simulink model "gm_CustArch_v13_vnl"  (R2020a)
settings: Solver=FixedStepDiscrete  StartTime=0.0  StopTime=840000  RelTol=1e-3
libraries: simulink x185, hdlsllib x109, hdlmdlgenlib x25, dsparch4 x1
(part 3 of 4)

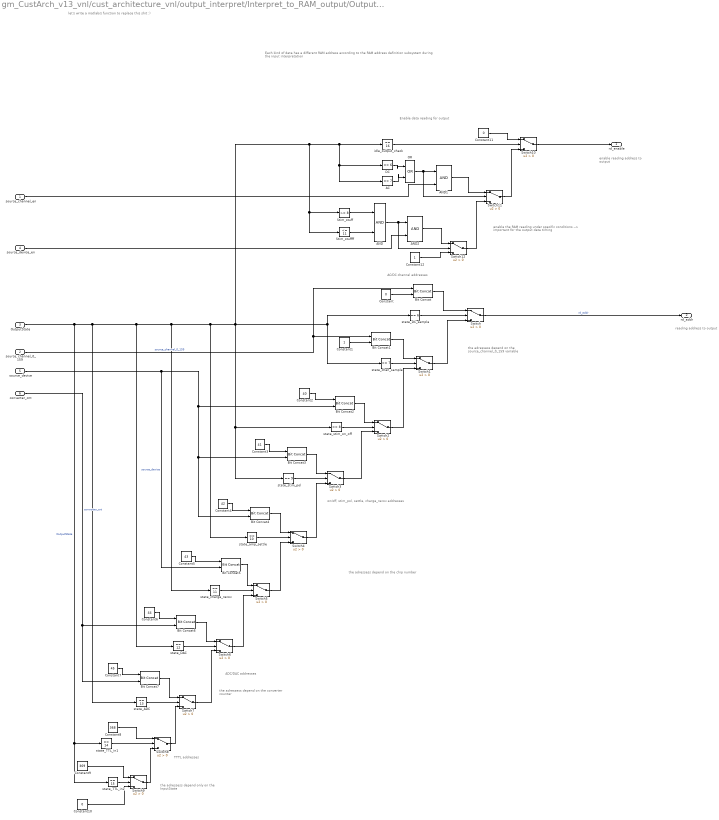
== system gm_CustArch_v13_vnl/cust_architecture_vnl/output_interpret/Interpret_to_RAM_output/Output_State_to_RAM_address (to read) ==
  note: enable reading address
      | to output
  note: Each kind of data has a different RAM
      | address according to the
      | RAM address definition subsystem during the
      | input interpretation
  note: the adressess depend on the
      | source_channel_0_159 variable
  note: AC/DC channel addresses
  note: ADC/DAC addresses
  note: on/off, stim_pol, settle, charge_recov addresses
  note: the adressess depend on the converter
      | counter
  note: the adressess depend only on the
      | InputState
  note: the adressess depend on the chip number
  note: TTTL addresses
  note: let's write a matlab/s function to replace this shit :)
  note: Enable data reading for output
  note: enable the RAM reading under specific conditions
      | --> important for the output data timing
  note: reading address
      | to output
  source_channel_en : Inport
  source_channel_0_159 : Inport  Port=2
  OutputState : Inport  Port=3
  source_device_en : Inport  Port=4
  source_device : Inport  Port=5
  converter_cnt : Inport  Port=6
  AC : simulink/Logic and Bit Operations/Compare To Constant  relop===  const=7  OutDataTypeStr=boolean
  AND : Logic  IconShape=distinctive  AllPortsSameDT=off  OutDataTypeStr=boolean
  AND1 : Logic  IconShape=distinctive  AllPortsSameDT=off  OutDataTypeStr=boolean
  AND2 : Logic  IconShape=distinctive  AllPortsSameDT=off  OutDataTypeStr=boolean
  Bit Concat{,1..7} (8 alike) : hdlsllib/Logic and Bit Operations/Bit Concat  numInputs=2
  Constant : Constant  Value=0  OutDataTypeStr=boolean  SampleTime=-1
  Constant1 : Constant  OutDataTypeStr=boolean  SampleTime=-1
  Constant10 : Constant  Value=0  OutDataTypeStr=fixdt(0,9)  SampleTime=-1
  Constant11 : Constant  Value=0  OutDataTypeStr=boolean  SampleTime=-1
  Constant12 : Constant  OutDataTypeStr=boolean  SampleTime=-1
  Constant2 : Constant  Value=40  OutDataTypeStr=fixdt(0,6)  SampleTime=-1
  Constant3 : Constant  Value=41  OutDataTypeStr=fixdt(0,6)  SampleTime=-1
  Constant4 : Constant  Value=42  OutDataTypeStr=fixdt(0,6)  SampleTime=-1
  Constant5 : Constant  Value=43  OutDataTypeStr=fixdt(0,6)  SampleTime=-1
  Constant6 : Constant  Value=44  OutDataTypeStr=fixdt(0,6)  SampleTime=-1
  Constant7 : Constant  Value=45  OutDataTypeStr=fixdt(0,6)  SampleTime=-1
  Constant8 : Constant  Value=368  OutDataTypeStr=fixdt(0,9)  SampleTime=-1
  Constant9 : Constant  Value=369  OutDataTypeStr=fixdt(0,9)  SampleTime=-1
  DC : simulink/Logic and Bit Operations/Compare To Constant  relop===  const=6  OutDataTypeStr=boolean
  OR : Logic  Operator=OR  IconShape=distinctive  AllPortsSameDT=off  OutDataTypeStr=boolean
  Stim_stuff : simulink/Logic and Bit Operations/Compare To Constant  relop=>=  const=8  OutDataTypeStr=boolean
  Stim_stuffff : simulink/Logic and Bit Operations/Compare To Constant  relop=<=  const=11  OutDataTypeStr=boolean
  Switch{,1..12} (13 alike) : Switch  Criteria=u2 > Threshold
  idle_output_check : simulink/Logic and Bit Operations/Compare To Constant  relop===  const=16  OutDataTypeStr=boolean
  state_ADC : simulink/Logic and Bit Operations/Compare To Constant  relop===  const=13  OutDataTypeStr=boolean
  state_DAC : simulink/Logic and Bit Operations/Compare To Constant  relop===  const=12  OutDataTypeStr=boolean
  state_DC_sample : simulink/Logic and Bit Operations/Compare To Constant  relop===  const=6  OutDataTypeStr=boolean
  state_TTL_in1 : simulink/Logic and Bit Operations/Compare To Constant  relop===  const=14  OutDataTypeStr=boolean
  state_TTL_in2 : simulink/Logic and Bit Operations/Compare To Constant  relop===  const=15  OutDataTypeStr=boolean
  state_amp_settle : simulink/Logic and Bit Operations/Compare To Constant  relop===  const=10  OutDataTypeStr=boolean
  state_chan_sample : simulink/Logic and Bit Operations/Compare To Constant  relop===  const=7  OutDataTypeStr=boolean
  state_charge_recov : simulink/Logic and Bit Operations/Compare To Constant  relop===  const=11  OutDataTypeStr=boolean
  state_stim_on_off : simulink/Logic and Bit Operations/Compare To Constant  relop===  const=8  OutDataTypeStr=boolean
  state_stim_pol : simulink/Logic and Bit Operations/Compare To Constant  relop===  const=9  OutDataTypeStr=boolean
  rd_enable : Outport  VectorParamsAs1DForOutWhenUnconnected=off
  rd_addr : Outport  Port=2  OutDataTypeStr=fixdt(0,9,0)  VectorParamsAs1DForOutWhenUnconnected=off
  wires:
  Switch10/1 -> rd_enable/1
  Constant12/1 -> Switch12/3
  Switch12/1 -> Switch11/3
  AND2/1 -> Switch12/1
  AND1/1 -> Switch11/1
  Switch11/1 -> Switch10/3
  Constant11/1 -> Switch10/1
  source_device_en/1 -> AND2/2
  source_channel_en/1 -> AND1/2
  AND/1 -> AND2/1, Switch12/2
  Stim_stuffff/1 -> AND/2
  Stim_stuff/1 -> AND/1
  idle_output_check/1 -> Switch10/2
  OR/1 -> AND1/1, Switch11/2
  AC/1 -> OR/2
  DC/1 -> OR/1
  Constant10/1 -> Switch9/3
  Switch9/1 -> Switch8/3
  Constant9/1 -> Switch9/1
  state_TTL_in2/1 -> Switch9/2
  Switch8/1 -> Switch7/3
  OutputState/1 -> state_ADC/1, state_charge_recov/1, Stim_stuff/1, Stim_stuffff/1, idle_output_check/1, DC/1, AC/1, state_chan_sample/1, state_DC_sample/1, state_stim_on_off/1, state_stim_pol/1, state_amp_settle/1, state_DAC/1, state_TTL_in1/1, state_TTL_in2/1  "OutputState"
  Constant8/1 -> Switch8/1
  state_TTL_in1/1 -> Switch8/2
  Switch7/1 -> Switch6/3
  Constant7/1 -> Bit Concat7/1
  state_ADC/1 -> Switch7/2
  Bit Concat7/1 -> Switch7/1
  converter_cnt/1 -> Bit Concat6/2, Bit Concat7/2  "converter_cnt"
  Switch6/1 -> Switch5/3
  Constant6/1 -> Bit Concat6/1
  state_DAC/1 -> Switch6/2
  Bit Concat6/1 -> Switch6/1
  Switch5/1 -> Switch4/3
  source_device/1 -> Bit Concat2/2, Bit Concat3/2, Bit Concat4/2, Bit Concat5/2  "source_device"
  Constant5/1 -> Bit Concat5/1
  state_charge_recov/1 -> Switch5/2
  Bit Concat5/1 -> Switch5/1
  Switch4/1 -> Switch3/3
  Bit Concat4/1 -> Switch4/1
  state_amp_settle/1 -> Switch4/2
  Constant4/1 -> Bit Concat4/1
  Switch3/1 -> Switch2/3
  Bit Concat3/1 -> Switch3/1
  state_stim_pol/1 -> Switch3/2
  Constant3/1 -> Bit Concat3/1
  Switch2/1 -> Switch1/3
  state_stim_on_off/1 -> Switch2/2
  Bit Concat2/1 -> Switch2/1
  Constant2/1 -> Bit Concat2/1
  Switch/1 -> rd_addr/1  "rd_addr"
  Switch1/1 -> Switch/3
  Bit Concat1/1 -> Switch1/1
  Constant1/1 -> Bit Concat1/2
  state_chan_sample/1 -> Switch1/2
  Bit Concat/1 -> Switch/1
  Constant/1 -> Bit Concat/2
  source_channel_0_159/1 -> Bit Concat/1, Bit Concat1/1  "source_channel_0_159"
  state_DC_sample/1 -> Switch/2

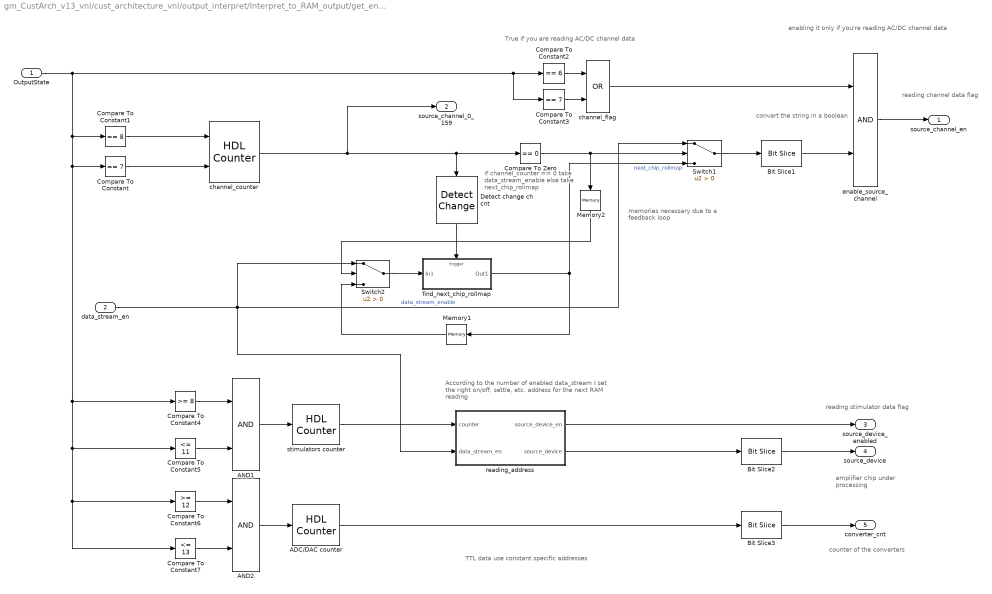
== system gm_CustArch_v13_vnl/cust_architecture_vnl/output_interpret/Interpret_to_RAM_output/get_enabled_timings  ==
  note: counter of the converters
  note: reading stimulator data flag
  note: TTL data use constant specific addresses
  note: enabling it only if you're reading AC/DC channel data
  note: True if you are reading AC/DC channel data
  note: convert the string
      | in a boolean
  note: According to the number of enabled data_stream
      | I set the right on/off, settle, etc. address for the next
      | RAM reading
  note: amplifier chip under
      | processing
  note: if channel_counter == 0
      | take data_stream_enable
      | else take next_chip_rollmap
  note: memories necessary due to
      | a feedback loop
  note: reading channel data flag
  OutputState : Inport
  data_stream_en : Inport  Port=2
  ADC/DAC counter : hdlsllib/Sources/HDL Counter  CountType=Count limited  CountInit=0  CountStep=1  CountMax=7  CountFromType=Specify  CountFrom=0  CountResetPort=off  CountLoadPort=off  CountEnbPort=on  CountDirPort=off  CountDataType=Unsigned  CountWordLen=8  CountFracLen=0  CountSampTime=1
  AND1 : Logic  IconShape=distinctive  AllPortsSameDT=off  OutDataTypeStr=boolean
  AND2 : Logic  IconShape=distinctive  AllPortsSameDT=off  OutDataTypeStr=boolean
  Bit Slice1 : hdlsllib/Logic and Bit Operations/Bit Slice  lidx=0  ridx=0
      settings: SourceProductBaseCode=SL
  Bit Slice2 : hdlsllib/Logic and Bit Operations/Bit Slice  lidx=2  ridx=0
      settings: SourceProductBaseCode=SL
  Bit Slice3 : hdlsllib/Logic and Bit Operations/Bit Slice  lidx=2  ridx=0
      settings: SourceProductBaseCode=SL
  Compare To Constant : simulink/Logic and Bit Operations/Compare To Constant  relop===  const=7  OutDataTypeStr=boolean
  Compare To Constant1 : simulink/Logic and Bit Operations/Compare To Constant  relop===  const=8  OutDataTypeStr=boolean
  Compare To Constant2 : simulink/Logic and Bit Operations/Compare To Constant  relop===  const=6  OutDataTypeStr=boolean
  Compare To Constant3 : simulink/Logic and Bit Operations/Compare To Constant  relop===  const=7  OutDataTypeStr=boolean
  Compare To Constant4 : simulink/Logic and Bit Operations/Compare To Constant  relop=>=  const=8  OutDataTypeStr=boolean
  Compare To Constant5 : simulink/Logic and Bit Operations/Compare To Constant  relop=<=  const=11  OutDataTypeStr=boolean
  Compare To Constant6 : simulink/Logic and Bit Operations/Compare To Constant  relop=>=  const=12  OutDataTypeStr=boolean
  Compare To Constant7 : simulink/Logic and Bit Operations/Compare To Constant  relop=<=  const=13  OutDataTypeStr=boolean
  Compare To Zero : simulink/Logic and Bit Operations/Compare To Zero  relop===  OutDataTypeStr=boolean
  Detect change ch cnt : simulink/Logic and Bit Operations/Detect Change  vinit=0  OutDataTypeStr=boolean
  Memory1 : Memory  InheritSampleTime=on
  Memory2 : Memory  InheritSampleTime=on
  Switch1 : Switch  Criteria=u2 > Threshold
  Switch2 : Switch  Criteria=u2 > Threshold
  channel_counter : hdlsllib/Sources/HDL Counter  CountType=Count limited  CountInit=0  CountStep=1  CountMax=159  CountFromType=Specify  CountFrom=0  CountResetPort=on  CountLoadPort=off  CountEnbPort=on  CountDirPort=off  CountDataType=Unsigned  CountWordLen=8  CountFracLen=0  CountSampTime=1
  channel_flag : Logic  Operator=OR  IconShape=distinctive  AllPortsSameDT=off  OutDataTypeStr=boolean
  enable_source_channel : Logic  IconShape=distinctive  AllPortsSameDT=off  OutDataTypeStr=boolean
  find_next_chip_rollmap : Subsystem  TreatAsAtomicUnit=on
  reading_address : Subsystem
  stimulators counter : hdlsllib/Sources/HDL Counter  CountType=Count limited  CountInit=0  CountStep=1  CountMax=7  CountFromType=Specify  CountFrom=0  CountResetPort=off  CountLoadPort=off  CountEnbPort=on  CountDirPort=off  CountDataType=Unsigned  CountWordLen=8  CountFracLen=0  CountSampTime=1
  source_channel_en : Outport  VectorParamsAs1DForOutWhenUnconnected=off
  source_channel_0_159 : Outport  Port=2  OutMin=0  OutMax=159  OutDataTypeStr=uint8  VectorParamsAs1DForOutWhenUnconnected=off  LockScale=on
  source_device_enabled : Outport  Port=3  VectorParamsAs1DForOutWhenUnconnected=off
  source_device : Outport  Port=4  VectorParamsAs1DForOutWhenUnconnected=off
  converter_cnt : Outport  Port=5  VectorParamsAs1DForOutWhenUnconnected=off
  wires:
  Compare To Constant/1 -> channel_counter/2
  Compare To Constant1/1 -> channel_counter/1
  ADC/DAC counter/1 -> Bit Slice3/1
  AND2/1 -> ADC/DAC counter/1
  Compare To Constant7/1 -> AND2/2
  OutputState/1 -> Compare To Constant2/1, Compare To Constant3/1, Compare To Constant4/1, Compare To Constant5/1, Compare To Constant7/1, Compare To Constant6/1, Compare To Constant/1, Compare To Constant1/1
  Bit Slice3/1 -> converter_cnt/1
  Compare To Constant6/1 -> AND2/1
  data_stream_en/1 -> Switch2/1, reading_address/2(data_stream_en), Switch1/1  "data_stream_enable"
  reading_address/2(source_device) -> Bit Slice2/1
  stimulators counter/1 -> reading_address/1("counter ")
  AND1/1 -> stimulators counter/1
  Bit Slice2/1 -> source_device/1
  reading_address/1(source_device_en) -> source_device_enabled/1
  Compare To Constant5/1 -> AND1/2
  Compare To Constant4/1 -> AND1/1
  Bit Slice1/1 -> enable_source_channel/2
  Switch1/1 -> Bit Slice1/1
  enable_source_channel/1 -> source_channel_en/1
  channel_flag/1 -> enable_source_channel/1
  Compare To Constant2/1 -> channel_flag/1
  Compare To Constant3/1 -> channel_flag/2
  Memory2/1 -> Switch2/2
  Compare To Zero/1 -> Memory2/1, Switch1/2
  Switch2/1 -> find_next_chip_rollmap/1(In1)
  Memory1/1 -> Switch2/3
  find_next_chip_rollmap/1(Out1) -> Switch1/3, Memory1/1  "next_chip_rollmap"
  Detect change ch cnt/1 -> find_next_chip_rollmap/Trigger
  channel_counter/1 -> source_channel_0_159/1, Compare To Zero/1, Detect change ch cnt/1

== system gm_CustArch_v13_vnl/cust_architecture_vnl/process_and_retrieve/Filter_ch1/digital_filter ==
  raw_input : Inport  OutDataTypeStr=uint16  LockScale=on
  Enable : EnablePort
  Add : Sum  Inputs=+-  OutDataTypeStr=fixdt(1,32,16)
  Add1 : Sum  OutDataTypeStr=fixdt(0,16,0)
  Constant : Constant  Value=32768  OutDataTypeStr=fixdt(0,16,0)  SampleTime=-1
  Constant1 : Constant  Value=32768  OutDataTypeStr=fixdt(0,16,0)  SampleTime=-1
  highpass : Subsystem  Tag=BlockMethodSubSystem
  filter_output : Outport  InitialOutput=[0]  LockScale=on
  wires:
  Add1/1 -> filter_output/1
  raw_input/1 -> Add/1
  highpass/1(Out) -> Add1/1
  Constant1/1 -> Add1/2
  Add/1 -> highpass/1(In)
  Constant/1 -> Add/2

== system gm_CustArch_v13_vnl/cust_architecture/input_interpret_store_retrieve/Interpret_to_RAM_input/interpret incoming data/condition to count DAC or ADC  ==
  fifo_write_to : Inport  OutDataTypeStr=boolean  PortDimensions=1  SampleTime=1
  input_state : Inport  Port=2  OutDataTypeStr=uint8  PortDimensions=1  SampleTime=1
  AND : Logic  AllPortsSameDT=off  OutDataTypeStr=boolean  SampleTime=1
  OR : Logic  Operator=OR  AllPortsSameDT=off  OutDataTypeStr=boolean  SampleTime=1
  is state_ADC : simulink/Logic and Bit Operations/Compare To Constant  relop===  const="fi(0,0,8,0,\"hex\",\"0d\")"  OutDataTypeStr=boolean
  is state_DAC : simulink/Logic and Bit Operations/Compare To Constant  relop===  const="fi(0,0,8,0,\"hex\",\"0c\")"  OutDataTypeStr=boolean
  Out1 : Outport  VectorParamsAs1DForOutWhenUnconnected=off
  wires:
  is state_DAC/1 -> OR/1
  is state_ADC/1 -> OR/2
  OR/1 -> AND/2
  AND/1 -> Out1/1
  input_state/1 -> is state_ADC/1, is state_DAC/1
  fifo_write_to/1 -> AND/1

== system gm_CustArch_v13_vnl/cust_architecture/input_interpret_store_retrieve/Interpret_to_RAM_input/interpret incoming data/get_sources_and_RAM_addresses ==
  note: necessary to move forward from state 6 to 8
  note: 0-159 --> 20 (16 electrodes + 4 aux commands) x 8 chips
  note: if next_chip_rollmap == 00000000 I have cycled among all the chip so let's restart from data_stream_enable
  note: the data_stream_enable is a 8-bit string in which if a bit is 1 the data stream of that chip is enabled
  note: TTL data use constant specific addresses
  FIFO_write_to : Inport  OutDataTypeStr=boolean  PortDimensions=1  SampleTime=1
  InputState : Inport  Port=2  OutDataTypeStr=uint8  PortDimensions=1  SampleTime=1
  data_stream_enable : Inport  Port=3  OutDataTypeStr=uint8  PortDimensions=1  SampleTime=1
  AND1 : Logic  AllPortsSameDT=off  OutDataTypeStr=boolean  SampleTime=1
  AND2 : Logic  AllPortsSameDT=off  OutDataTypeStr=boolean  SampleTime=1
  AND3 : Logic  AllPortsSameDT=off  OutDataTypeStr=boolean  SampleTime=1
  Compare To Constant1 : simulink/Logic and Bit Operations/Compare To Constant  relop===  const="fi(0,0,8,0,\"hex\",\"00\")"  OutDataTypeStr=boolean
  Compare To Constant2 : simulink/Logic and Bit Operations/Compare To Constant  relop===  const="fi(0,0,8,0,\"hex\",\"0d\")"  OutDataTypeStr=boolean
  Compare To Constant3 : simulink/Logic and Bit Operations/Compare To Constant  relop===  const="fi(0,0,8,0,\"hex\",\"06\")"  OutDataTypeStr=boolean
  Compare To Constant4 : simulink/Logic and Bit Operations/Compare To Constant  relop=>=  const="fi(0,0,8,0,\"hex\",\"08\")"  OutDataTypeStr=boolean
  Compare To Constant5 : simulink/Logic and Bit Operations/Compare To Constant  relop===  const="fi(0,0,8,0,\"hex\",\"00\")"  OutDataTypeStr=boolean
  Compare To Constant6 : simulink/Logic and Bit Operations/Compare To Constant  relop=<=  const="fi(0,0,8,0,\"hex\",\"0b\")"  OutDataTypeStr=boolean
  Memory : UnitDelay  InitialCondition=double(0)  SampleTime=1
  Memory1 : UnitDelay  InitialCondition=double(0)  SampleTime=1
  Memory2 : UnitDelay  InitialCondition=double(0)  SampleTime=1
  OR : Logic  Operator=OR  AllPortsSameDT=off  OutDataTypeStr=boolean  SampleTime=1
  RAM_address_channel_data : Subsystem
  Switch : Switch  Criteria=u2 > Threshold  Threshold=double(0)  OutDataTypeStr=uint8  SampleTime=1
  Switch1 : Switch  Criteria=u2 > Threshold  Threshold=double(0)  OutDataTypeStr=uint8  SampleTime=1
  channel_counter : hdlsllib/Sources/HDL Counter  CountType=Count limited  CountInit=double(0)  CountStep=double(1)  CountMax=double(20)  CountFromType=Initial value  CountFrom=double(0)  CountResetPort=on  CountLoadPort=off  CountEnbPort=on  CountDirPort=off  CountDataType=Unsigned  CountWordLen=8  CountFracLen=0  CountSampTime=1
  enable_RAM_indexing : Logic  AllPortsSameDT=off  OutDataTypeStr=boolean  SampleTime=1
  enable_source_chip_transmission : Subsystem
  find_first_one_pos : Subsystem
  find_next_chip_rollmap : Subsystem
  source_device : Outport  VectorParamsAs1DForOutWhenUnconnected=off
  device_output : Outport  Port=2  VectorParamsAs1DForOutWhenUnconnected=off
  source_channel : Outport  Port=3  VectorParamsAs1DForOutWhenUnconnected=off
  inc_source_device : Outport  Port=4  VectorParamsAs1DForOutWhenUnconnected=off
  wires:
  find_next_chip_rollmap/1(bit_masked) -> Memory/1, Compare To Constant5/1
  find_first_one_pos/1(first_one_pos) -> find_next_chip_rollmap/2(source_chip), enable_source_chip_transmission/1(In1)
  enable_source_chip_transmission/1(Out1) -> RAM_address_channel_data/1(source_device), source_device/1
  enable_RAM_indexing/1 -> find_first_one_pos/Enable, find_next_chip_rollmap/Enable, RAM_address_channel_data/Enable, enable_source_chip_transmission/Enable, Memory2/1, AND2/1
  channel_counter/1 -> RAM_address_channel_data/2(dev_output), device_output/1
  Switch1/1 -> Switch/3
  Switch/1 -> find_first_one_pos/1(In1), find_next_chip_rollmap/1(curr_chip_rollmap)
  RAM_address_channel_data/1(source_channel_0_159) -> source_channel/1
  OR/1 -> enable_RAM_indexing/2
  Memory2/1 -> AND3/2
  Memory1/1 -> AND3/1, Switch1/2
  Memory/1 -> Switch1/3
  Compare To Constant6/1 -> AND1/2
  Compare To Constant5/1 -> Memory1/1, AND2/2
  Compare To Constant4/1 -> AND1/1
  Compare To Constant3/1 -> OR/1
  Compare To Constant2/1 -> channel_counter/1
  Compare To Constant1/1 -> Switch/2
  AND3/1 -> channel_counter/2
  AND2/1 -> inc_source_device/1
  AND1/1 -> OR/2
  data_stream_enable/1 -> Switch/1, Switch1/1
  InputState/1 -> Compare To Constant1/1, Compare To Constant2/1, Compare To Constant3/1, Compare To Constant4/1, Compare To Constant6/1
  FIFO_write_to/1 -> enable_RAM_indexing/1

== system gm_CustArch_v13_vnl/cust_architecture/output_interpret/Interpret_to_RAM_output/get_enabled_timings /find_next_chip_rollmap ==
  In1 : Inport  OutDataTypeStr=uint8  PortDimensions=1
  Trigger : TriggerPort  VariantControl=(inherit)  PortDimensions=1  OutDataTypeStr=boolean
  Bit Rotate : hdlsllib/Logic and Bit Operations/Bit Rotate  mode=Rotate Right  N=double(1)
      settings: SourceProductBaseCode=SL
  Out1 : Outport  InitialOutput=0  VectorParamsAs1DForOutWhenUnconnected=off
  wires:
  Bit Rotate/1 -> Out1/1
  In1/1 -> Bit Rotate/1

== system gm_CustArch_v13_vnl/cust_architecture/output_interpret/Interpret_to_RAM_output/get_enabled_timings /reading_address ==
  "counter " : Inport  OutDataTypeStr=uint8  PortDimensions=1  SampleTime=1
  data_stream_en : Inport  Port=2  OutDataTypeStr=uint8  PortDimensions=1  SampleTime=1
  Bit Rotate : hdlsllib/Logic and Bit Operations/Bit Rotate  mode=Rotate Right  N=double(1)
      settings: SourceProductBaseCode=SL
  Bit Rotate1 : hdlsllib/Logic and Bit Operations/Bit Rotate  mode=Rotate Right  N=double(2)
      settings: SourceProductBaseCode=SL
  Bit Rotate2 : hdlsllib/Logic and Bit Operations/Bit Rotate  mode=Rotate Right  N=double(3)
      settings: SourceProductBaseCode=SL
  Bit Rotate3 : hdlsllib/Logic and Bit Operations/Bit Rotate  mode=Rotate Right  N=double(4)
      settings: SourceProductBaseCode=SL
  Bit Rotate4 : hdlsllib/Logic and Bit Operations/Bit Rotate  mode=Rotate Right  N=double(5)
      settings: SourceProductBaseCode=SL
  Bit Rotate5 : hdlsllib/Logic and Bit Operations/Bit Rotate  mode=Rotate Right  N=double(6)
      settings: SourceProductBaseCode=SL
  Bit Rotate6 : hdlsllib/Logic and Bit Operations/Bit Rotate  mode=Rotate Right  N=double(7)
      settings: SourceProductBaseCode=SL
  Bit Slice : hdlsllib/Logic and Bit Operations/Bit Slice  lidx=double(0)  ridx=double(0)
      settings: SourceProductBaseCode=SL
  Compare To Constant : simulink/Logic and Bit Operations/Compare To Constant  relop===  const="fi(0,0,8,0,\"hex\",\"00\")"  OutDataTypeStr=boolean
  Compare To Constant1 : simulink/Logic and Bit Operations/Compare To Constant  relop===  const="fi(0,0,8,0,\"hex\",\"01\")"  OutDataTypeStr=boolean
  Compare To Constant2 : simulink/Logic and Bit Operations/Compare To Constant  relop===  const="fi(0,0,8,0,\"hex\",\"02\")"  OutDataTypeStr=boolean
  Compare To Constant3 : simulink/Logic and Bit Operations/Compare To Constant  relop===  const="fi(0,0,8,0,\"hex\",\"03\")"  OutDataTypeStr=boolean
  Compare To Constant4 : simulink/Logic and Bit Operations/Compare To Constant  relop===  const="fi(0,0,8,0,\"hex\",\"04\")"  OutDataTypeStr=boolean
  Compare To Constant5 : simulink/Logic and Bit Operations/Compare To Constant  relop===  const="fi(0,0,8,0,\"hex\",\"05\")"  OutDataTypeStr=boolean
  Compare To Constant6 : simulink/Logic and Bit Operations/Compare To Constant  relop===  const="fi(0,0,8,0,\"hex\",\"06\")"  OutDataTypeStr=boolean
  Compare To Constant7 : simulink/Logic and Bit Operations/Compare To Constant  relop===  const="fi(0,0,8,0,\"hex\",\"07\")"  OutDataTypeStr=boolean
  Constant : Constant  Value=0  OutDataTypeStr=uint8  SampleTime=1
  Switch{,1..7} (8 alike) : Switch  Criteria=u2 > Threshold  Threshold=double(0)  OutDataTypeStr=uint8  SampleTime=1
  source_device_en : Outport  VectorParamsAs1DForOutWhenUnconnected=off
  source_device : Outport  Port=2  VectorParamsAs1DForOutWhenUnconnected=off
  wires:
  Switch7/1 -> Switch6/3
  Switch6/1 -> Switch5/3
  Switch5/1 -> Switch4/3
  Switch4/1 -> Switch3/3
  Switch3/1 -> Switch2/3
  Switch2/1 -> Switch1/3
  Switch1/1 -> Switch/3
  Switch/1 -> Bit Slice/1
  Constant/1 -> Switch7/3
  Compare To Constant7/1 -> Switch7/2
  Compare To Constant6/1 -> Switch6/2
  Compare To Constant5/1 -> Switch5/2
  Compare To Constant4/1 -> Switch4/2
  Compare To Constant3/1 -> Switch3/2
  Compare To Constant2/1 -> Switch2/2
  Compare To Constant1/1 -> Switch1/2
  Compare To Constant/1 -> Switch/2
  Bit Slice/1 -> source_device_en/1
  Bit Rotate6/1 -> Switch7/1
  Bit Rotate5/1 -> Switch6/1
  Bit Rotate4/1 -> Switch5/1
  Bit Rotate3/1 -> Switch4/1
  Bit Rotate2/1 -> Switch3/1
  Bit Rotate1/1 -> Switch2/1
  Bit Rotate/1 -> Switch1/1
  data_stream_en/1 -> Bit Rotate/1, Bit Rotate1/1, Bit Rotate2/1, Bit Rotate3/1, Bit Rotate4/1, Bit Rotate5/1, Bit Rotate6/1, Switch/1
  "counter "/1 -> source_device/1, Compare To Constant/1, Compare To Constant1/1, Compare To Constant2/1, Compare To Constant3/1, Compare To Constant4/1, Compare To Constant5/1, Compare To Constant6/1, Compare To Constant7/1

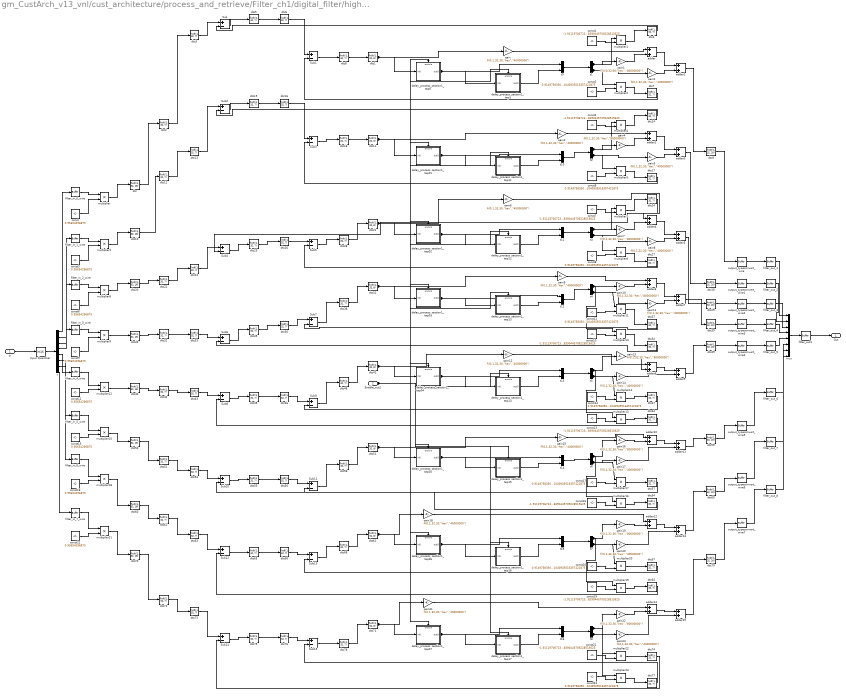
== system gm_CustArch_v13_vnl/cust_architecture/process_and_retrieve/Filter_ch1/digital_filter/highpass ==
  In : Inport  OutDataTypeStr=fixdt(1, 32, 16)  PortDimensions=[8 1]  SampleTime=1
  Enable_out2 : Inport  Port=2  OutDataTypeStr=boolean  SampleTime=1
  Input Quantizer : DataTypeConversion  OutDataTypeStr=int16  RndMeth=Round  SampleTime=1  SaturateOnIntegerOverflow=on
  Sub{,1..15} (16 alike) : Sum  Inputs=+-  OutDataTypeStr=fixdt(1, 33, 7)  RndMeth=Nearest  SaturateOnIntegerOverflow=on  SampleTime=1
  adder{,1..15} (16 alike) : Sum  OutDataTypeStr=fixdt(1, 32, 7)  RndMeth=Nearest  SaturateOnIntegerOverflow=on  SampleTime=1
  const{,3,6,9,12,15,18,21} (8 alike) : Constant  Value=0.95654296875  OutDataTypeStr=fixdt(1, 32, 15)  SampleTime=1
  const{1,4,7,10,13,16,19,22} (8 alike) : Constant  Value=-1.911197067238390445709228515625  OutDataTypeStr=fixdt(1, 32, 30)  SampleTime=1
  const{2,5,8,11,14,17,20,23} (8 alike) : Constant  Value=0.91497583501040935516357421875  OutDataTypeStr=fixdt(1, 32, 30)  SampleTime=1
  delay_process_section1_tap0 : Subsystem
      settings: MinAlgLoopOccurrences=on
  delay_process_section1_tap01 : Subsystem
      settings: MinAlgLoopOccurrences=on
  delay_process_section1_tap02 : Subsystem
      settings: MinAlgLoopOccurrences=on
  delay_process_section1_tap03 : Subsystem
      settings: MinAlgLoopOccurrences=on
  delay_process_section1_tap04 : Subsystem
      settings: MinAlgLoopOccurrences=on
  delay_process_section1_tap05 : Subsystem
      settings: MinAlgLoopOccurrences=on
  delay_process_section1_tap06 : Subsystem
      settings: MinAlgLoopOccurrences=on
  delay_process_section1_tap07 : Subsystem
      settings: MinAlgLoopOccurrences=on
  delay_process_section1_tap1 : Subsystem
      settings: MinAlgLoopOccurrences=on
  delay_process_section1_tap11 : Subsystem
      settings: MinAlgLoopOccurrences=on
  delay_process_section1_tap12 : Subsystem
      settings: MinAlgLoopOccurrences=on
  delay_process_section1_tap13 : Subsystem
      settings: MinAlgLoopOccurrences=on
  delay_process_section1_tap14 : Subsystem
      settings: MinAlgLoopOccurrences=on
  delay_process_section1_tap15 : Subsystem
      settings: MinAlgLoopOccurrences=on
  delay_process_section1_tap16 : Subsystem
      settings: MinAlgLoopOccurrences=on
  delay_process_section1_tap17 : Subsystem
      settings: MinAlgLoopOccurrences=on
  dtc{,10,20,30,40,50,60,70} (8 alike) : DataTypeConversion  OutDataTypeStr=fixdt(1, 32, 16)  RndMeth=Nearest  SampleTime=1  SaturateOnIntegerOverflow=on
  dtc{1,11,21,31,41,51,61,71} (8 alike) : DataTypeConversion  OutDataTypeStr=fixdt(1, 32, 8)  RndMeth=Nearest  SampleTime=1  SaturateOnIntegerOverflow=on
  dtc{2,12,22,32,42,52,62,72} (8 alike) : DataTypeConversion  OutDataTypeStr=fixdt(1, 32, 7)  RndMeth=Nearest  SampleTime=1  SaturateOnIntegerOverflow=on
  dtc{3..8,13..18,23..28,33..38,43..48,53..58,63..68,73..78} (48 alike) : DataTypeConversion  OutDataTypeStr=fixdt(1, 32, 7)  RndMeth=Nearest  SampleTime=1
  dtc{9,19,29,39,49,59,69,79} (8 alike) : DataTypeConversion  OutDataTypeStr=fixdt(1, 32, 20)  RndMeth=Nearest  SampleTime=1  SaturateOnIntegerOverflow=on
  filter_in_0_wire : hdlmdlgenlib/Buffer
      settings: SourceProductBaseCode=SL
  filter_in_1_wire : hdlmdlgenlib/Buffer
      settings: SourceProductBaseCode=SL
  filter_in_2_wire : hdlmdlgenlib/Buffer
      settings: SourceProductBaseCode=SL
  filter_in_3_wire : hdlmdlgenlib/Buffer
      settings: SourceProductBaseCode=SL
  filter_in_4_wire : hdlmdlgenlib/Buffer
      settings: SourceProductBaseCode=SL
  filter_in_5_wire : hdlmdlgenlib/Buffer
      settings: SourceProductBaseCode=SL
  filter_in_6_wire : hdlmdlgenlib/Buffer
      settings: SourceProductBaseCode=SL
  filter_in_7_wire : hdlmdlgenlib/Buffer
      settings: SourceProductBaseCode=SL
  filter_out1 : hdlmdlgenlib/Buffer
      settings: SourceProductBaseCode=SL
  filter_out_{1..8} (8 alike) : hdlmdlgenlib/Buffer
      settings: SourceProductBaseCode=SL
  gain{,2..3,5..6,8..9,11..12,14..15,17..18,20..21,23} (16 alike) : Gain  Gain="fi(0,1,32,30,\"hex\",\"40000000\")"  ParamDataTypeStr=fixdt(1, 32, 30)  OutDataTypeStr=fixdt(1, 32, 7)  RndMeth=Nearest  SampleTime=1
  gain{1,4,7,10,13,16,19,22} (8 alike) : Gain  Gain="fi(0,1,32,30,\"hex\",\"80000000\")"  ParamDataTypeStr=fixdt(1, 32, 30)  OutDataTypeStr=fixdt(1, 32, 7)  RndMeth=Nearest  SampleTime=1
  multiplier{,3,6,9,12,15,18,21} (8 alike) : Product  Inputs=**  OutDataTypeStr=fixdt(1, 64, 26)  RndMeth=Nearest  SampleTime=1
  multiplier{1..2,4..5,7..8,10..11,13..14,16..17,19..20,22..23} (16 alike) : Product  Inputs=**  OutDataTypeStr=fixdt(1, 32, 7)  RndMeth=Nearest  SampleTime=1
  mux : Mux  Inputs=8
  output_typeconvert_wire{,1..7} (8 alike) : hdlmdlgenlib/Buffer
      settings: SourceProductBaseCode=SL
  t : Demux  Outputs=8
  t{1..8} (8 alike) : Demux  Outputs=2
  t{9..16} (8 alike) : Mux  Inputs=2
  Out : Outport  InitialOutput=0
  wires:
  Enable_out2/1 -> delay_process_section1_tap0/Enable, delay_process_section1_tap1/Enable, delay_process_section1_tap01/Enable, delay_process_section1_tap11/Enable, delay_process_section1_tap02/Enable, delay_process_section1_tap12/Enable, delay_process_section1_tap03/Enable, delay_process_section1_tap13/Enable, delay_process_section1_tap04/Enable, delay_process_section1_tap14/Enable, delay_process_section1_tap05/Enable, delay_process_section1_tap15/Enable, delay_process_section1_tap06/Enable, delay_process_section1_tap16/Enable, delay_process_section1_tap07/Enable, delay_process_section1_tap17/Enable
  delay_process_section1_tap17/1(out0) -> t16/2
  delay_process_section1_tap07/1(out0) -> t16/1, delay_process_section1_tap17/1(in0)
  delay_process_section1_tap16/1(out0) -> t15/2
  delay_process_section1_tap06/1(out0) -> t15/1, delay_process_section1_tap16/1(in0)
  delay_process_section1_tap15/1(out0) -> t14/2
  delay_process_section1_tap05/1(out0) -> t14/1, delay_process_section1_tap15/1(in0)
  delay_process_section1_tap14/1(out0) -> t13/2
  delay_process_section1_tap04/1(out0) -> t13/1, delay_process_section1_tap14/1(in0)
  delay_process_section1_tap13/1(out0) -> t12/2
  delay_process_section1_tap03/1(out0) -> t12/1, delay_process_section1_tap13/1(in0)
  delay_process_section1_tap12/1(out0) -> t11/2
  delay_process_section1_tap02/1(out0) -> t11/1, delay_process_section1_tap12/1(in0)
  delay_process_section1_tap11/1(out0) -> t10/2
  delay_process_section1_tap01/1(out0) -> t10/1, delay_process_section1_tap11/1(in0)
  delay_process_section1_tap1/1(out0) -> t9/2
  delay_process_section1_tap0/1(out0) -> t9/1, delay_process_section1_tap1/1(in0)
  dtc79/1 -> output_typeconvert_wire7/1
  Sub15/1 -> dtc78/1
  dtc77/1 -> Sub15/2
  dtc76/1 -> Sub15/1
  Sub14/1 -> dtc75/1
  dtc74/1 -> Sub14/2
  dtc73/1 -> Sub14/1
  gain23/1 -> adder15/2
  gain22/1 -> adder14/2
  gain21/1 -> adder14/1
  multiplier23/1 -> dtc77/1
  multiplier22/1 -> dtc74/1
  dtc72/1 -> dtc73/1
  t8/2 -> multiplier23/1, gain23/1
  t8/1 -> multiplier22/1, gain22/1
  t16/1 -> t8/1
  dtc71/1 -> gain21/1, delay_process_section1_tap07/1(in0)
  adder14/1 -> adder15/1
  adder15/1 -> dtc79/1
  dtc75/1 -> dtc76/1
  dtc78/1 -> dtc71/1
  dtc70/1 -> dtc72/1
  const23/1 -> multiplier23/2
  const22/1 -> multiplier22/2
  multiplier21/1 -> dtc70/1
  const21/1 -> multiplier21/2
  output_typeconvert_wire7/1 -> filter_out_8/1
  dtc69/1 -> output_typeconvert_wire6/1
  Sub13/1 -> dtc68/1
  dtc67/1 -> Sub13/2
  dtc66/1 -> Sub13/1
  Sub12/1 -> dtc65/1
  dtc64/1 -> Sub12/2
  dtc63/1 -> Sub12/1
  gain20/1 -> adder13/2
  gain19/1 -> adder12/2
  gain18/1 -> adder12/1
  multiplier20/1 -> dtc67/1
  multiplier19/1 -> dtc64/1
  dtc62/1 -> dtc63/1
  t7/2 -> gain20/1, multiplier20/1
  t7/1 -> gain19/1, multiplier19/1
  t15/1 -> t7/1
  dtc61/1 -> gain18/1, delay_process_section1_tap06/1(in0)
  adder12/1 -> adder13/1
  adder13/1 -> dtc69/1
  dtc65/1 -> dtc66/1
  dtc68/1 -> dtc61/1
  dtc60/1 -> dtc62/1
  const20/1 -> multiplier20/2
  const19/1 -> multiplier19/2
  multiplier18/1 -> dtc60/1
  const18/1 -> multiplier18/2
  output_typeconvert_wire6/1 -> filter_out_7/1
  dtc59/1 -> output_typeconvert_wire5/1
  Sub11/1 -> dtc58/1
  dtc57/1 -> Sub11/2
  dtc56/1 -> Sub11/1
  Sub10/1 -> dtc55/1
  dtc54/1 -> Sub10/2
  dtc53/1 -> Sub10/1
  gain17/1 -> adder11/2
  gain16/1 -> adder10/2
  gain15/1 -> adder10/1
  multiplier17/1 -> dtc57/1
  multiplier16/1 -> dtc54/1
  dtc52/1 -> dtc53/1
  t6/2 -> gain17/1, multiplier17/1
  t6/1 -> gain16/1, multiplier16/1
  t14/1 -> t6/1
  dtc51/1 -> gain15/1, delay_process_section1_tap05/1(in0)
  adder10/1 -> adder11/1
  adder11/1 -> dtc59/1
  dtc55/1 -> dtc56/1
  dtc58/1 -> dtc51/1
  dtc50/1 -> dtc52/1
  const17/1 -> multiplier17/2
  const16/1 -> multiplier16/2
  multiplier15/1 -> dtc50/1
  const15/1 -> multiplier15/2
  output_typeconvert_wire5/1 -> filter_out_6/1
  dtc49/1 -> output_typeconvert_wire4/1
  Sub9/1 -> dtc48/1
  dtc47/1 -> Sub9/2
  dtc46/1 -> Sub9/1
  Sub8/1 -> dtc45/1
  dtc44/1 -> Sub8/2
  dtc43/1 -> Sub8/1
  gain14/1 -> adder9/2
  gain13/1 -> adder8/2
  gain12/1 -> adder8/1
  multiplier14/1 -> dtc47/1
  multiplier13/1 -> dtc44/1
  dtc42/1 -> dtc43/1
  t5/2 -> gain14/1, multiplier14/1
  t5/1 -> gain13/1, multiplier13/1
  t13/1 -> t5/1
  dtc41/1 -> gain12/1, delay_process_section1_tap04/1(in0)
  adder8/1 -> adder9/1
  adder9/1 -> dtc49/1
  dtc45/1 -> dtc46/1
  dtc48/1 -> dtc41/1
  dtc40/1 -> dtc42/1
  const14/1 -> multiplier14/2
  const13/1 -> multiplier13/2
  multiplier12/1 -> dtc40/1
  const12/1 -> multiplier12/2
  output_typeconvert_wire4/1 -> filter_out_5/1
  dtc39/1 -> output_typeconvert_wire3/1
  Sub7/1 -> dtc38/1
  dtc37/1 -> Sub7/2
  dtc36/1 -> Sub7/1
  Sub6/1 -> dtc35/1
  dtc34/1 -> Sub6/2
  dtc33/1 -> Sub6/1
  gain11/1 -> adder7/2
  gain10/1 -> adder6/2
  gain9/1 -> adder6/1
  multiplier11/1 -> dtc37/1
  multiplier10/1 -> dtc34/1
  dtc32/1 -> dtc33/1
  t4/2 -> gain11/1, multiplier11/1
  t4/1 -> gain10/1, multiplier10/1
  t12/1 -> t4/1
  dtc31/1 -> gain9/1, delay_process_section1_tap03/1(in0)
  adder6/1 -> adder7/1
  adder7/1 -> dtc39/1
  dtc35/1 -> dtc36/1
  dtc38/1 -> dtc31/1
  dtc30/1 -> dtc32/1
  const11/1 -> multiplier11/2
  const10/1 -> multiplier10/2
  multiplier9/1 -> dtc30/1
  const9/1 -> multiplier9/2
  output_typeconvert_wire3/1 -> filter_out_4/1
  dtc29/1 -> output_typeconvert_wire2/1
  Sub5/1 -> dtc28/1
  dtc27/1 -> Sub5/2
  dtc26/1 -> Sub5/1
  Sub4/1 -> dtc25/1
  dtc24/1 -> Sub4/2
  dtc23/1 -> Sub4/1
  gain8/1 -> adder5/2
  gain7/1 -> adder4/2
  gain6/1 -> adder4/1
  multiplier8/1 -> dtc27/1
  multiplier7/1 -> dtc24/1
  dtc22/1 -> dtc23/1
  t3/2 -> gain8/1, multiplier8/1
  t3/1 -> gain7/1, multiplier7/1
  t11/1 -> t3/1
  dtc21/1 -> gain6/1, delay_process_section1_tap02/1(in0)
  adder4/1 -> adder5/1
  adder5/1 -> dtc29/1
  dtc25/1 -> dtc26/1
  dtc28/1 -> dtc21/1
  dtc20/1 -> dtc22/1
  const8/1 -> multiplier8/2
  const7/1 -> multiplier7/2
  multiplier6/1 -> dtc20/1
  const6/1 -> multiplier6/2
  output_typeconvert_wire2/1 -> filter_out_3/1
  dtc19/1 -> output_typeconvert_wire1/1
  Sub3/1 -> dtc18/1
  dtc17/1 -> Sub3/2
  dtc16/1 -> Sub3/1
  Sub2/1 -> dtc15/1
  dtc14/1 -> Sub2/2
  dtc13/1 -> Sub2/1
  gain5/1 -> adder3/2
  gain4/1 -> adder2/2
  gain3/1 -> adder2/1
  multiplier5/1 -> dtc17/1
  multiplier4/1 -> dtc14/1
  dtc12/1 -> dtc13/1
  t2/2 -> gain5/1, multiplier5/1
  t2/1 -> gain4/1, multiplier4/1
  t10/1 -> t2/1
  dtc11/1 -> gain3/1, delay_process_section1_tap01/1(in0)
  adder2/1 -> adder3/1
  adder3/1 -> dtc19/1
  dtc15/1 -> dtc16/1
  dtc18/1 -> dtc11/1
  dtc10/1 -> dtc12/1
  const5/1 -> multiplier5/2
  const4/1 -> multiplier4/2
  multiplier3/1 -> dtc10/1
  const3/1 -> multiplier3/2
  output_typeconvert_wire1/1 -> filter_out_2/1
  dtc9/1 -> output_typeconvert_wire/1
  Sub1/1 -> dtc8/1
  dtc7/1 -> Sub1/2
  dtc6/1 -> Sub1/1
  Sub/1 -> dtc5/1
  dtc4/1 -> Sub/2
  dtc3/1 -> Sub/1
  gain2/1 -> adder1/2
  gain1/1 -> adder/2
  gain/1 -> adder/1
  multiplier2/1 -> dtc7/1
  multiplier1/1 -> dtc4/1
  dtc2/1 -> dtc3/1
  t1/2 -> gain2/1, multiplier2/1
  t1/1 -> gain1/1, multiplier1/1
  t9/1 -> t1/1
  dtc1/1 -> gain/1, delay_process_section1_tap0/1(in0)
  adder/1 -> adder1/1
  adder1/1 -> dtc9/1
  dtc5/1 -> dtc6/1
  dtc8/1 -> dtc1/1
  dtc/1 -> dtc2/1
  const2/1 -> multiplier2/2
  const1/1 -> multiplier1/2
  multiplier/1 -> dtc/1
  const/1 -> multiplier/2
  output_typeconvert_wire/1 -> filter_out_1/1
  t/8 -> filter_in_7_wire/1
  t/7 -> filter_in_6_wire/1
  t/6 -> filter_in_5_wire/1
  t/5 -> filter_in_4_wire/1
  t/4 -> filter_in_3_wire/1
  t/3 -> filter_in_2_wire/1
  t/2 -> filter_in_1_wire/1
  t/1 -> filter_in_0_wire/1
  filter_out_8/1 -> mux/8
  filter_in_7_wire/1 -> multiplier21/1
  filter_out_7/1 -> mux/7
  filter_in_6_wire/1 -> multiplier18/1
  filter_out_6/1 -> mux/6
  filter_in_5_wire/1 -> multiplier15/1
  filter_out_5/1 -> mux/5
  filter_in_4_wire/1 -> multiplier12/1
  filter_out_4/1 -> mux/4
  filter_in_3_wire/1 -> multiplier9/1
  filter_out_3/1 -> mux/3
  filter_in_2_wire/1 -> multiplier6/1
  filter_out_2/1 -> mux/2
  filter_in_1_wire/1 -> multiplier3/1
  filter_out_1/1 -> mux/1
  filter_in_0_wire/1 -> multiplier/1
  mux/1 -> filter_out1/1
  filter_out1/1 -> Out/1
  Input Quantizer/1 -> t/1
  In/1 -> Input Quantizer/1

== system gm_CustArch_v13_vnl/cust_architecture_vnl/input_interpret_store_retrieve/Interpret_to_RAM_input/interpret incoming data/condition to count DAC or ADC  ==
  fifo_write_to : Inport
  input_state : Inport  Port=2
  AND : Logic  IconShape=distinctive  AllPortsSameDT=off  OutDataTypeStr=boolean
  OR : Logic  Operator=OR  IconShape=distinctive  AllPortsSameDT=off  OutDataTypeStr=boolean
  is state_ADC : simulink/Logic and Bit Operations/Compare To Constant  relop===  const=13  OutDataTypeStr=boolean
  is state_DAC : simulink/Logic and Bit Operations/Compare To Constant  relop===  const=12  OutDataTypeStr=boolean
  Out1 : Outport  VectorParamsAs1DForOutWhenUnconnected=off
  wires:
  AND/1 -> Out1/1
  OR/1 -> AND/2
  fifo_write_to/1 -> AND/1
  is state_ADC/1 -> OR/2
  is state_DAC/1 -> OR/1
  input_state/1 -> is state_ADC/1, is state_DAC/1

== system gm_CustArch_v13_vnl/cust_architecture_vnl/input_interpret_store_retrieve/Interpret_to_RAM_input/interpret incoming data/get_sources_and_RAM_addresses ==
  note: TTL data use constant specific addresses
  note: channel data
      | address
  note: channel (electrode) under
      | processing
  note: the data_stream_enable is a 8-bit string in which if a bit is 1 the data stream of that chip is enabled
  note: if next_chip_rollmap == 00000000 I have cycled among all the chip so let's restart from data_stream_enable
  note: to identify the first position in which
      | I am able to find a 1
  note: 0-159 --> 20 (16 electrodes + 4 aux commands) x 8 chips
  note: if InputState == 0 (starting state corresponding to the first byte
      | of the magic number) the data_stream_enable goes through the switch
  note: whether or not enable the address definition
      | for the RAM writing
  note: if InputState == 13
      | reset the channel counter
  note: the channel_counter increments the
      | device_output variable every time the
      | current_chip rollmap is equal to 00000000
      | (rollmap concluded)
  note: amplifier chip under
      | processing
  note: necessary to move forward from state 6 to 8
  FIFO_write_to : Inport
  InputState : Inport  Port=2
  data_stream_enable : Inport  Port=3
  AND1 : Logic  IconShape=distinctive  AllPortsSameDT=off  OutDataTypeStr=boolean
  AND2 : Logic  IconShape=distinctive  AllPortsSameDT=off  OutDataTypeStr=boolean
  AND3 : Logic  IconShape=distinctive  AllPortsSameDT=off  OutDataTypeStr=boolean
  Compare To Constant1 : simulink/Logic and Bit Operations/Compare To Constant  relop===  const=0  OutDataTypeStr=boolean
  Compare To Constant2 : simulink/Logic and Bit Operations/Compare To Constant  relop===  const=13  OutDataTypeStr=boolean
  Compare To Constant3 : simulink/Logic and Bit Operations/Compare To Constant  relop===  const=6  OutDataTypeStr=boolean
  Compare To Constant4 : simulink/Logic and Bit Operations/Compare To Constant  relop=>=  const=8  OutDataTypeStr=boolean
  Compare To Constant5 : simulink/Logic and Bit Operations/Compare To Constant  relop===  const=0  OutDataTypeStr=boolean
  Compare To Constant6 : simulink/Logic and Bit Operations/Compare To Constant  relop=<=  const=11  OutDataTypeStr=boolean
  Memory : Memory  InheritSampleTime=on
  Memory1 : Memory  InheritSampleTime=on
  Memory2 : Memory  InheritSampleTime=on
  OR : Logic  Operator=OR  IconShape=distinctive  AllPortsSameDT=off  OutDataTypeStr=boolean
  RAM_address_channel_data : Subsystem
  Switch : Switch  Criteria=u2 > Threshold  OutDataTypeStr=uint8
  Switch1 : Switch  Criteria=u2 > Threshold
  channel_counter : hdlsllib/Sources/HDL Counter  CountType=Count limited  CountInit=0  CountStep=1  CountMax=20  CountFromType=Specify  CountFrom=0  CountResetPort=on  CountLoadPort=off  CountEnbPort=on  CountDirPort=off  CountDataType=Unsigned  CountWordLen=8  CountFracLen=0  CountSampTime=1
  enable_RAM_indexing : Logic  IconShape=distinctive  AllPortsSameDT=off  OutDataTypeStr=boolean
  enable_source_chip_transmission : Subsystem  TreatAsAtomicUnit=on
  find_first_one_pos : Subsystem
  find_next_chip_rollmap : Subsystem
  source_device : Outport  VectorParamsAs1DForOutWhenUnconnected=off
  device_output : Outport  Port=2  VectorParamsAs1DForOutWhenUnconnected=off
  source_channel : Outport  Port=3  VectorParamsAs1DForOutWhenUnconnected=off
  inc_source_device : Outport  Port=4  VectorParamsAs1DForOutWhenUnconnected=off
  wires:
  find_first_one_pos/1(first_one_pos) -> find_next_chip_rollmap/2(source_chip), enable_source_chip_transmission/1(In1)  "source_device"
  AND2/1 -> inc_source_device/1
  Memory1/1 -> Switch1/2, AND3/1
  OR/1 -> enable_RAM_indexing/2
  AND1/1 -> OR/2
  Compare To Constant6/1 -> AND1/2
  Compare To Constant4/1 -> AND1/1
  Compare To Constant2/1 -> channel_counter/1
  RAM_address_channel_data/1(source_channel_0_159) -> source_channel/1  "source_channel_0_159"
  Compare To Constant3/1 -> OR/1
  enable_source_chip_transmission/1(Out1) -> RAM_address_channel_data/1(source_device), source_device/1  "source_device"
  Memory2/1 -> AND3/2
  Memory/1 -> Switch1/3
  AND3/1 -> channel_counter/2
  channel_counter/1 -> RAM_address_channel_data/2(dev_output), device_output/1  "device_output"
  Compare To Constant5/1 -> Memory1/1, AND2/2
  Switch1/1 -> Switch/3
  enable_RAM_indexing/1 -> AND2/1, Memory2/1, find_first_one_pos/Enable, find_next_chip_rollmap/Enable, RAM_address_channel_data/Enable, enable_source_chip_transmission/Enable
  FIFO_write_to/1 -> enable_RAM_indexing/1
  find_next_chip_rollmap/1(bit_masked) -> Compare To Constant5/1, Memory/1  "next_chip_rollmap"
  data_stream_enable/1 -> Switch/1, Switch1/1
  Compare To Constant1/1 -> Switch/2
  Switch/1 -> find_first_one_pos/1(In1), find_next_chip_rollmap/1(curr_chip_rollmap)  "curr_chip_rollmap"
  InputState/1 -> Compare To Constant3/1, Compare To Constant4/1, Compare To Constant6/1, Compare To Constant2/1, Compare To Constant1/1  "input state"

== system gm_CustArch_v13_vnl/cust_architecture_vnl/output_interpret/Interpret_to_RAM_output/get_enabled_timings /find_next_chip_rollmap ==
  note: bit rotation --> circular rotation of the data_stream_enable 8-bit string
      |
      | Example: data_stream_enable == 01001000
      | right rotation length 1 --> 00100100
      | right rotation length 3 --> 10000100
  note: this is to identify the next chip for decoding process
  In1 : Inport
  Trigger : TriggerPort  VariantControl=Variant
  Bit Rotate : hdlsllib/Logic and Bit Operations/Bit Rotate  mode=Rotate Right  N=1
      settings: SourceProductBaseCode=SL
  Out1 : Outport  InitialOutput=0  VectorParamsAs1DForOutWhenUnconnected=off
  wires:
  Bit Rotate/1 -> Out1/1
  In1/1 -> Bit Rotate/1

== system gm_CustArch_v13_vnl/cust_architecture_vnl/output_interpret/Interpret_to_RAM_output/get_enabled_timings /reading_address ==
  note: this is the ugliest thing ever--- but it works.. so far so good
  "counter " : Inport
  data_stream_en : Inport  Port=2
  Bit Rotate : hdlsllib/Logic and Bit Operations/Bit Rotate  mode=Rotate Right  N=1
      settings: SourceProductBaseCode=SL
  Bit Rotate1 : hdlsllib/Logic and Bit Operations/Bit Rotate  mode=Rotate Right  N=2
      settings: SourceProductBaseCode=SL
  Bit Rotate2 : hdlsllib/Logic and Bit Operations/Bit Rotate  mode=Rotate Right  N=3
      settings: SourceProductBaseCode=SL
  Bit Rotate3 : hdlsllib/Logic and Bit Operations/Bit Rotate  mode=Rotate Right  N=4
      settings: SourceProductBaseCode=SL
  Bit Rotate4 : hdlsllib/Logic and Bit Operations/Bit Rotate  mode=Rotate Right  N=5
      settings: SourceProductBaseCode=SL
  Bit Rotate5 : hdlsllib/Logic and Bit Operations/Bit Rotate  mode=Rotate Right  N=6
      settings: SourceProductBaseCode=SL
  Bit Rotate6 : hdlsllib/Logic and Bit Operations/Bit Rotate  mode=Rotate Right  N=7
      settings: SourceProductBaseCode=SL
  Bit Slice : hdlsllib/Logic and Bit Operations/Bit Slice  lidx=0  ridx=0
      settings: SourceProductBaseCode=SL
  Compare To Constant : simulink/Logic and Bit Operations/Compare To Constant  relop===  const=0  OutDataTypeStr=boolean
  Compare To Constant1 : simulink/Logic and Bit Operations/Compare To Constant  relop===  const=1  OutDataTypeStr=boolean
  Compare To Constant2 : simulink/Logic and Bit Operations/Compare To Constant  relop===  const=2  OutDataTypeStr=boolean
  Compare To Constant3 : simulink/Logic and Bit Operations/Compare To Constant  relop===  const=3  OutDataTypeStr=boolean
  Compare To Constant4 : simulink/Logic and Bit Operations/Compare To Constant  relop===  const=4  OutDataTypeStr=boolean
  Compare To Constant5 : simulink/Logic and Bit Operations/Compare To Constant  relop===  const=5  OutDataTypeStr=boolean
  Compare To Constant6 : simulink/Logic and Bit Operations/Compare To Constant  relop===  const=6  OutDataTypeStr=boolean
  Compare To Constant7 : simulink/Logic and Bit Operations/Compare To Constant  relop===  const=7  OutDataTypeStr=boolean
  Constant : Constant  Value=0  OutDataTypeStr=uint8  SampleTime=-1
  Switch{,1..7} (8 alike) : Switch  Criteria=u2 > Threshold
  source_device_en : Outport  VectorParamsAs1DForOutWhenUnconnected=off
  source_device : Outport  Port=2  VectorParamsAs1DForOutWhenUnconnected=off
  wires:
  Bit Slice/1 -> source_device_en/1
  Switch/1 -> Bit Slice/1
  data_stream_en/1 -> Bit Rotate6/1, Bit Rotate5/1, Bit Rotate4/1, Bit Rotate3/1, Bit Rotate2/1, Bit Rotate1/1, Bit Rotate/1, Switch/1
  Switch2/1 -> Switch1/3
  Constant/1 -> Switch7/3
  Bit Rotate6/1 -> Switch7/1
  Switch7/1 -> Switch6/3
  Compare To Constant7/1 -> Switch7/2
  Bit Rotate5/1 -> Switch6/1
  Switch6/1 -> Switch5/3
  Compare To Constant6/1 -> Switch6/2
  Switch5/1 -> Switch4/3
  Bit Rotate4/1 -> Switch5/1
  Compare To Constant5/1 -> Switch5/2
  Bit Rotate3/1 -> Switch4/1
  Switch4/1 -> Switch3/3
  Compare To Constant4/1 -> Switch4/2
  Bit Rotate2/1 -> Switch3/1
  Switch3/1 -> Switch2/3
  Compare To Constant3/1 -> Switch3/2
  Bit Rotate1/1 -> Switch2/1
  Compare To Constant2/1 -> Switch2/2
  Switch1/1 -> Switch/3
  "counter "/1 -> source_device/1, Compare To Constant/1, Compare To Constant1/1, Compare To Constant2/1, Compare To Constant3/1, Compare To Constant4/1, Compare To Constant5/1, Compare To Constant6/1, Compare To Constant7/1
  Bit Rotate/1 -> Switch1/1
  Compare To Constant1/1 -> Switch1/2
  Compare To Constant/1 -> Switch/2

== system gm_CustArch_v13_vnl/cust_architecture_vnl/process_and_retrieve/Filter_ch1/digital_filter/highpass ==
  In : Inport  OutDataTypeStr=fixdt(1,32,16)
  Input Quantizer : DataTypeConversion  OutDataTypeStr=fixdt(1,16,0)  RndMeth=Round  SaturateOnIntegerOverflow=on
  filter : dsparch4/Biquad Filter  FilterSource=Dialog parameters  CoeffSource=Specify via dialog  FilterObject=BQF  IIRFiltStruct=Direct form II  BiQuadCoeffs=[1 -2 1 1 -1.9111970674260732 0.914975834801433852]  ScaleValues=[0.956543225556876764;1]  IC=0  ICnum=0  ICden=0  a0Flag=Warning  optimizeScaleValues=on  ScaleValueMode=Specify via input port (g)  roundingMode=Nearest  overflowMode=on  stageInputMode=Binary point scaling  stageInputWordLength=32  stageInputFracLength=16  stageOutputMode=Binary point scaling  stageOutputWordLength=32  stageOutputFracLength=11  firstCoeffMode=Binary point scaling  firstCoeffWordLength=32  firstCoeffFracLength=30  scaleValueFracLength=15  prodOutputMode=Binary point scaling  prodOutputWordLength=32  prodOutputFracLength=7  denProdOutputFracLength=7  accumMode=Binary point scaling  accumWordLength=32  accumFracLength=7  denAccumFracLength=7  memoryMode=Binary point scaling  memoryWordLength=32  memoryFracLength=8  secondMemoryFracLength=15  outputMode=Binary point scaling  outputWordLength=32  outputFracLength=20
  Out : Outport
  wires:
  filter/1 -> Out/1
  Input Quantizer/1 -> filter/1
  In/1 -> Input Quantizer/1

== system gm_CustArch_v13_vnl/cust_architecture/input_interpret_store_retrieve/Interpret_to_RAM_input/interpret incoming data/get_sources_and_RAM_addresses/RAM_address_channel_data ==
  source_device : Inport  OutDataTypeStr=uint8  PortDimensions=1  SampleTime=1
  dev_output : Inport  Port=2  OutDataTypeStr=uint8  PortDimensions=1  SampleTime=1
  Enable : EnablePort  OutDataTypeStr=boolean
  Bit Concat : hdlsllib/Logic and Bit Operations/Bit Concat  numInputs=2
  Bit Slice : hdlsllib/Logic and Bit Operations/Bit Slice  lidx=double(4)  ridx=double(0)
      settings: SourceProductBaseCode=SL
  Bit Slice1 : hdlsllib/Logic and Bit Operations/Bit Slice  lidx=double(2)  ridx=double(0)
      settings: SourceProductBaseCode=SL
  source_channel_0_159 : Outport  InitialOutput=0  VectorParamsAs1DForOutWhenUnconnected=off
  wires:
  Bit Slice1/1 -> Bit Concat/2
  Bit Slice/1 -> Bit Concat/1
  Bit Concat/1 -> source_channel_0_159/1
  dev_output/1 -> Bit Slice/1
  source_device/1 -> Bit Slice1/1

== system gm_CustArch_v13_vnl/cust_architecture/input_interpret_store_retrieve/Interpret_to_RAM_input/interpret incoming data/get_sources_and_RAM_addresses/enable_source_chip_transmission ==
  In1 : Inport  OutDataTypeStr=uint8  PortDimensions=1  SampleTime=1
  Enable : EnablePort  OutDataTypeStr=boolean
  Out1 : Outport  InitialOutput=0  VectorParamsAs1DForOutWhenUnconnected=off
  wires:
  In1/1 -> Out1/1
